simulink library "rr_general"  (R2018b)
settings: Solver=VariableStepAuto  StartTime=0.0  StopTime=10.0  RelTol=1e-3  EnableMultiTasking=on
undefined symbols (not defined in the file): DiscIntNeverNeededParam, P_MLOC_OSS_FrontX, P_MLOC_OSS_FrontY, tPX2CommsTimeout
libraries: simulink x4
settings Model: Creator=wischnewski  LastModifiedBy=ge34qer
settings OptimizationCC: LifeSpan=inf
settings SFSimCC: SimUseLocalCustomCode=off
settings RTWCC: RTWUseLocalCustomCode=off
settings CodeAppCC: StateflowObjectComments=on

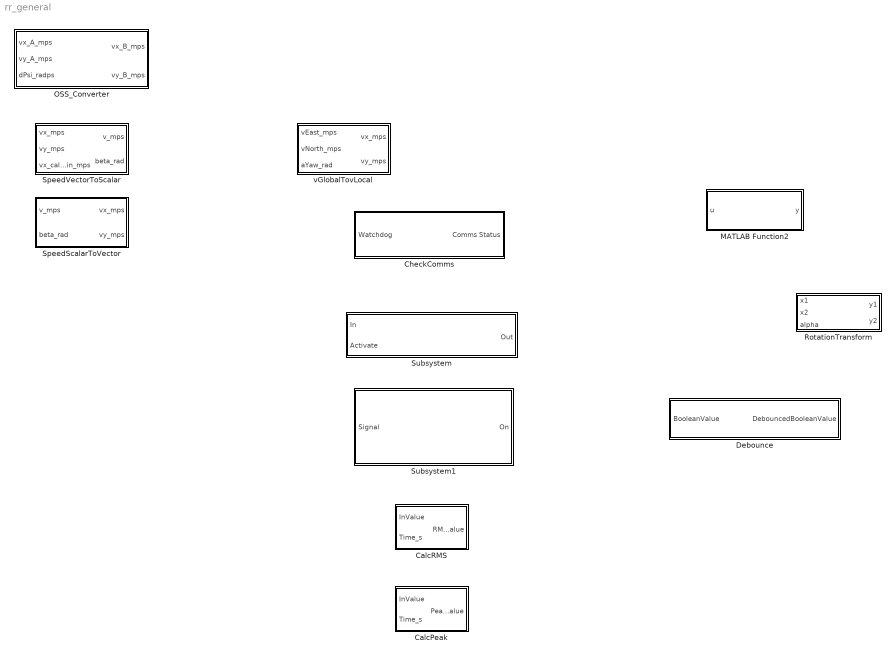
== system rr_general ==
  CalcPeak : Subsystem
  CalcRMS : Subsystem
  CheckComms : Subsystem  mask{timeout_s=0, tS=0}
      mask prompts: timeout_s "Timeout in s"; tS "Sample Time in s"
      mask DialogControl DescGroupVar Prompt: Block description
      mask DialogControl DescTextVar Prompt: Evaluates the communication status corresponding to the watchdog present at the input. If there is no change in the watchdog value detected for the timeout time, the communciation status is set to fail.
  Debounce : Subsystem  mask{debounce_cycles=0}
      mask prompts: debounce_cycles "Debounce cycles"
      mask DialogControl DebounceTitle Prompt: Debounce
      mask DialogControl DebounceText Prompt: Debounces the input signal for the given number of samples
  MATLAB Function2 : MATLAB Function  TreatAsAtomicUnit=on
  OSS_Converter : Subsystem
  RotationTransform : Subsystem
  SpeedScalarToVector : MATLAB Function  TreatAsAtomicUnit=on
  SpeedVectorToScalar : MATLAB Function  TreatAsAtomicUnit=on
  Subsystem : Subsystem  mask{UpperLimit=0, LowerLimit=0}
      mask prompts: UpperLimit "Upper bound for input signal"; LowerLimit "Lower bound for input signal"
      mask DialogControl Container4 Prompt: Description
      mask DialogControl Control2 Prompt: This block applies the limits specified at the bottom to the input signal. Furthermore, it only activates the output if the second input signal is a boolean which is true.
      mask Display:
      | disp('Limitation&\nActivation');
      | port_label('input', 1, 'Signal In');
      | port_label('input', 2, 'Active');
      | port_label('output', 1, 'Signal Out');
  Subsystem1 : Subsystem  mask{waitTime=0, Threshold=0}
      mask prompts: waitTime "Time until output is set to on"
      mask help: This block outputs true if the input signal is higher than the specified threshold for longer than the specified time.
      mask Display:
      | disp(['Wait until signal is \non for ' ' sec']);
      | port_label('input', 1, 'Signal In');
      | port_label('output', 1, 'On');
  vGlobalTovLocal : MATLAB Function  TreatAsAtomicUnit=on

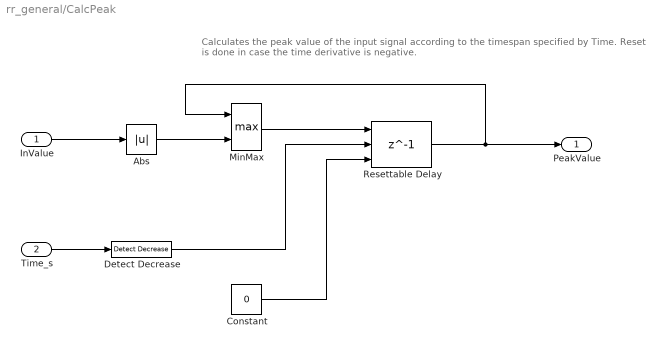
== system rr_general/CalcPeak ==
  note: Calculates the peak value of the input signal according to the timespan specified by Time.
      | Reset is done in case the time derivative is negative.
  InValue : Inport
  Time_s : Inport  Port=2
  Abs : Abs
  Constant : Constant  Value=0
  Detect Decrease : simulink/Logic and Bit Operations/Detect Decrease  vinit=0.0  OutDataTypeStr=boolean
  MinMax : MinMax  Function=max  Inputs=2
  Resettable Delay : Delay  DelayLength=1  InitialConditionSource=Input port  ExternalReset=Rising
      settings: InputPortMap=u0,r5,p4
  PeakValue : Outport
  wires:
  Time_s/1 -> Detect Decrease/1
  Resettable Delay/1 -> PeakValue/1, MinMax/1
  InValue/1 -> Abs/1
  Abs/1 -> MinMax/2
  MinMax/1 -> Resettable Delay/1
  Detect Decrease/1 -> Resettable Delay/2
  Constant/1 -> Resettable Delay/3

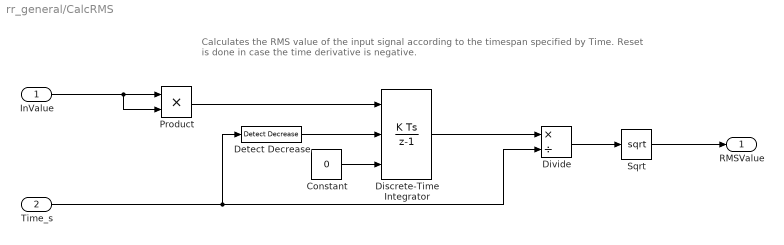
== system rr_general/CalcRMS ==
  note: Calculates the RMS value of the input signal according to the timespan specified by Time.
      | Reset is done in case the time derivative is negative.
  InValue : Inport
  Time_s : Inport  Port=2
  Constant : Constant  Value=0
  Detect Decrease : simulink/Logic and Bit Operations/Detect Decrease  vinit=0.0  OutDataTypeStr=boolean
  Discrete-Time Integrator : DiscreteIntegrator  ExternalReset=rising  InitialConditionSource=external  SampleTime=-1  ICPrevOutput=DiscIntNeverNeededParam  ICPrevScaledInput=DiscIntNeverNeededParam
  Divide : Product  Inputs=*/
  Product : Product
  Sqrt : Sqrt  SaturateOnIntegerOverflow=on
  RMSValue : Outport
  wires:
  Time_s/1 -> Detect Decrease/1, Divide/2
  Divide/1 -> Sqrt/1
  Discrete-Time Integrator/1 -> Divide/1
  Product/1 -> Discrete-Time Integrator/1
  Sqrt/1 -> RMSValue/1
  Detect Decrease/1 -> Discrete-Time Integrator/2
  InValue/1 -> Product/2, Product/1
  Constant/1 -> Discrete-Time Integrator/3

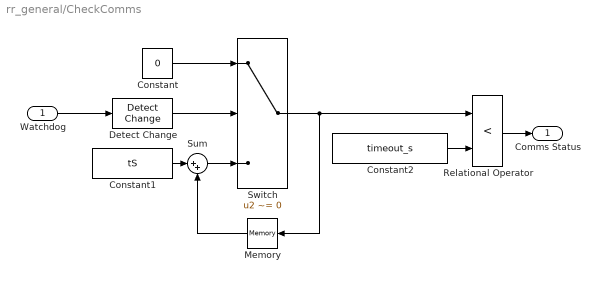
== system rr_general/CheckComms ==
  Watchdog : Inport
  Constant : Constant  Value=0
  Constant1 : Constant  Value=tS
  Constant2 : Constant  Value=timeout_s
  Detect Change : simulink/Logic and Bit Operations/Detect Change  vinit=0  OutDataTypeStr=boolean
  Memory : Memory  InitialCondition=tPX2CommsTimeout  InheritSampleTime=on
  Relational Operator : RelationalOperator  Operator=<  OutDataTypeStr=boolean  RndMeth=Nearest
  Sum : Sum  Inputs=|++
  Switch : Switch  Criteria=u2 ~= 0
  Comms Status : Outport
  wires:
  Watchdog/1 -> Detect Change/1
  Constant/1 -> Switch/1
  Switch/1 -> Relational Operator/1, Memory/1
  Constant1/1 -> Sum/1
  Sum/1 -> Switch/3
  Memory/1 -> Sum/2
  Detect Change/1 -> Switch/2
  Relational Operator/1 -> Comms Status/1
  Constant2/1 -> Relational Operator/2

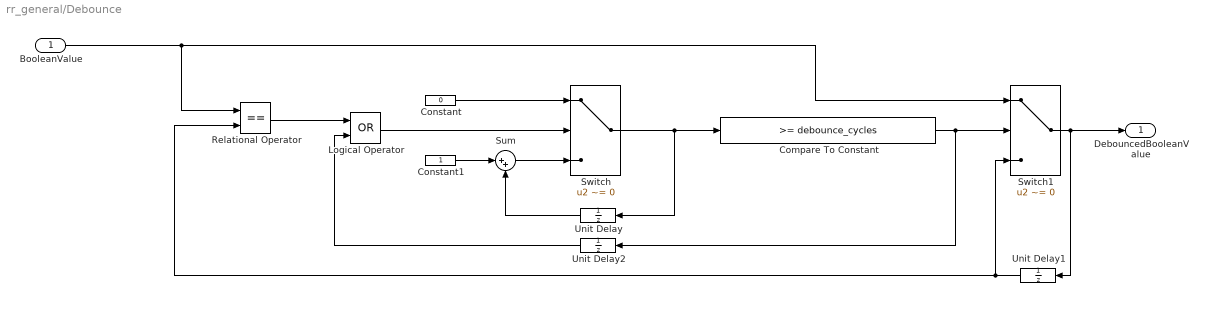
== system rr_general/Debounce ==
  BooleanValue : Inport  OutDataTypeStr=boolean
  Compare To Constant : simulink/Logic and Bit Operations/Compare To Constant  relop=>=  const=debounce_cycles  OutDataTypeStr=boolean
  Constant : Constant  Value=0
  Constant1 : Constant
  Logical Operator : Logic  Operator=OR  AllPortsSameDT=off  OutDataTypeStr=boolean
  Relational Operator : RelationalOperator  Operator===  OutDataTypeStr=boolean  RndMeth=Nearest
  Sum : Sum  Inputs=|++
  Switch : Switch  Criteria=u2 ~= 0
  Switch1 : Switch  Criteria=u2 ~= 0
  Unit Delay : UnitDelay  SampleTime=-1
  Unit Delay1 : UnitDelay  SampleTime=-1
  Unit Delay2 : UnitDelay  SampleTime=-1
  DebouncedBooleanValue : Outport  OutDataTypeStr=boolean
  wires:
  Constant1/1 -> Sum/1
  Unit Delay/1 -> Sum/2
  Sum/1 -> Switch/3
  Constant/1 -> Switch/1
  Switch/1 -> Unit Delay/1, Compare To Constant/1
  Compare To Constant/1 -> Unit Delay2/1, Switch1/2
  BooleanValue/1 -> Switch1/1, Relational Operator/1
  Unit Delay1/1 -> Switch1/3, Relational Operator/2
  Switch1/1 -> Unit Delay1/1, DebouncedBooleanValue/1
  Relational Operator/1 -> Logical Operator/1
  Logical Operator/1 -> Switch/2
  Unit Delay2/1 -> Logical Operator/2

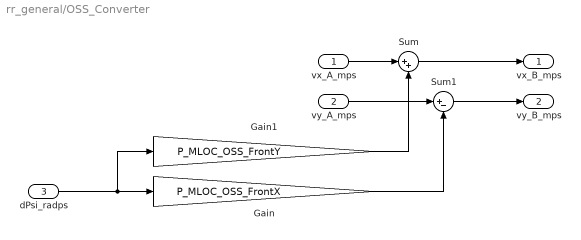
== system rr_general/OSS_Converter ==
  vx_A_mps : Inport
  vy_A_mps : Inport  Port=2
  dPsi_radps : Inport  Port=3
  Gain : Gain  Gain=P_MLOC_OSS_FrontX
  Gain1 : Gain  Gain=P_MLOC_OSS_FrontY
  Sum : Sum  Inputs=|++
  Sum1 : Sum  Inputs=|+-
  vx_B_mps : Outport
  vy_B_mps : Outport  Port=2
  wires:
  Gain/1 -> Sum1/2
  vy_A_mps/1 -> Sum1/1
  Gain1/1 -> Sum/2
  Sum/1 -> vx_B_mps/1
  Sum1/1 -> vy_B_mps/1
  vx_A_mps/1 -> Sum/1
  dPsi_radps/1 -> Gain1/1, Gain/1

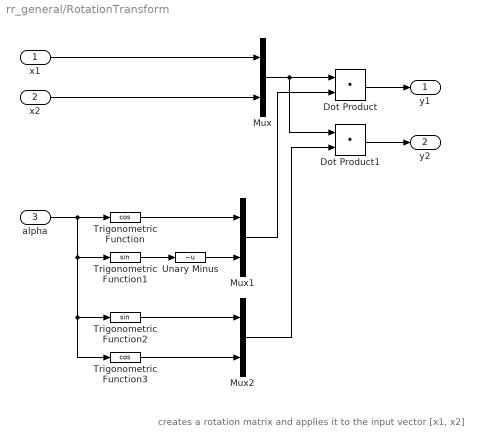
== system rr_general/RotationTransform ==
  note: creates a rotation matrix and applies it to the input vector [x1, x2]
  x1 : Inport
  x2 : Inport  Port=2
  alpha : Inport  Port=3
  Dot Product : DotProduct  InputSameDT=on  OutDataTypeStr=Inherit: Inherit via internal rule
  Dot Product1 : DotProduct  InputSameDT=on  OutDataTypeStr=Inherit: Inherit via internal rule
  Mux : Mux  Inputs=2
  Mux1 : Mux  Inputs=2
  Mux2 : Mux  Inputs=2
  Trigonometric Function : Trigonometry  Operator=cos
  Trigonometric Function1 : Trigonometry
  Trigonometric Function2 : Trigonometry
  Trigonometric Function3 : Trigonometry  Operator=cos
  Unary Minus : UnaryMinus
  y1 : Outport
  y2 : Outport  Port=2
  wires:
  x1/1 -> Mux/1
  x2/1 -> Mux/2
  Trigonometric Function/1 -> Mux1/1
  alpha/1 -> Trigonometric Function3/1, Trigonometric Function2/1, Trigonometric Function1/1, Trigonometric Function/1
  Trigonometric Function1/1 -> Unary Minus/1
  Trigonometric Function2/1 -> Mux2/1
  Trigonometric Function3/1 -> Mux2/2
  Unary Minus/1 -> Mux1/2
  Mux/1 -> Dot Product1/1, Dot Product/1
  Mux1/1 -> Dot Product/2
  Mux2/1 -> Dot Product1/2
  Dot Product/1 -> y1/1
  Dot Product1/1 -> y2/1

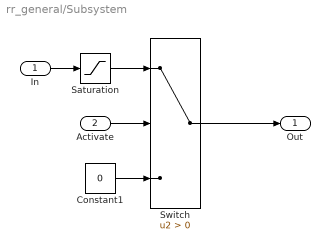
== system rr_general/Subsystem ==
  In : Inport
  Activate : Inport  Port=2  OutDataTypeStr=boolean
  Constant1 : Constant  Value=0
  Saturation : Saturate  UpperLimit=UpperLimit  LowerLimit=LowerLimit
  Switch : Switch  Criteria=u2 > Threshold
  Out : Outport
  wires:
  Constant1/1 -> Switch/3
  Switch/1 -> Out/1
  Activate/1 -> Switch/2
  Saturation/1 -> Switch/1
  In/1 -> Saturation/1

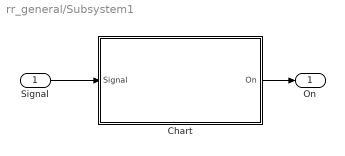
== system rr_general/Subsystem1 ==
  Signal : Inport
  Chart : Stateflow chart  TreatAsAtomicUnit=on
  On : Outport
  wires:
  Signal/1 -> Chart/1(Signal)
  Chart/1(On) -> On/1

== matlab function rr_general/SpeedScalarToVector ==
  data: v_mps input; vx_mps output; beta_rad input; vy_mps output
function [vx_mps, vy_mps] = fcn(v_mps, beta_rad)

[vx_mps, vy_mps] = vbeta2vxvy(v_mps, beta_rad); 

end

== matlab function rr_general/SpeedVectorToScalar ==
  data: vx_mps input; v_mps output; vy_mps input; beta_rad output; vx_calc_min_mps input
function [v_mps, beta_rad] = fcn(vx_mps, vy_mps, vx_calc_min_mps)

[v_mps, beta_rad] = vxvy2vbeta(vx_mps, vy_mps, vx_calc_min_mps); 

end

== stateflow chart rr_general/Subsystem1/Chart ==
  state WaitForCondition
    entry: On = false;
  state ConditionTrue
    state wait
    state ActivateOutput
      entry:
      On = true;
    (default) -> wait
    wait -> ActivateOutput : after(waitTime, sec)
  (default) -> WaitForCondition
  WaitForCondition -> ConditionTrue : [Signal >= Threshold]
  ConditionTrue -> WaitForCondition : [Signal < Threshold]
  data: Signal input; On output boolean; Threshold parameter; waitTime parameter

== matlab function rr_general/vGlobalTovLocal ==
  data: vEast_mps input; vx_mps output; vy_mps output; vNorth_mps input; aYaw_rad input
function [vx_mps, vy_mps] = fcn(vEast_mps, vNorth_mps, aYaw_rad)

  [vx_mps, vy_mps] = vGlobal2vLocal(vEast_mps, vNorth_mps, aYaw_rad);

end

== matlab function rr_general/MATLAB Function2 ==
  data: u input; y output
function y = normalizeAngle(u)

y = normalizeAngle(u);
